simulink model "rst_deadzone_example"  (R2014b)
settings: Solver=ode45  StartTime=0.0  StopTime=20  RelTol=1e-3
undefined symbols (not defined in the file): a1, a2, a3, b1, b2, b3, ea, h, r1, r2, r3, s0, s1, s2, t0
settings Model: Creator=Administrador  LastModifiedBy=kjartan

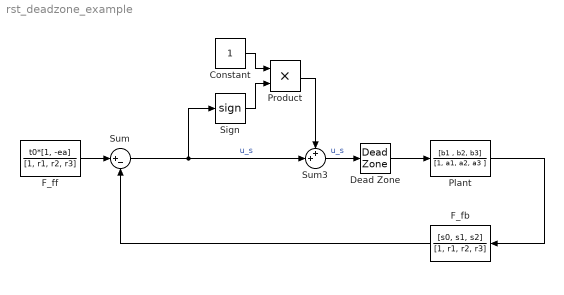
== system rst_deadzone_example ==
  Constant : Constant
  Dead Zone : DeadZone  LowerValue=-1  UpperValue=1  SaturateOnIntegerOverflow=on
  F_fb : DiscreteTransferFcn  Numerator=[s0, s1, s2]  Denominator=[1, r1, r2, r3]  SampleTime=h
  F_ff : DiscreteTransferFcn  Numerator=t0*[1, -ea]  Denominator=[1, r1, r2, r3]  SampleTime=h
  Plant : DiscreteTransferFcn  Numerator=[b1 , b2, b3]  Denominator=[1, a1, a2, a3 ]  SampleTime=h
  Product : Product
  Sign : Signum
  Sum : Sum  Inputs=|+-
  Sum3 : Sum  Inputs=++|
  wires:
  Plant/1 -> F_fb/1
  Sum/1 -> Sign/1, Sum3/2  "u_s"
  Constant/1 -> Product/1
  Sign/1 -> Product/2
  Product/1 -> Sum3/1
  Sum3/1 -> Dead Zone/1  "u_s"
  Dead Zone/1 -> Plant/1
  F_ff/1 -> Sum/1
  F_fb/1 -> Sum/2
